simulink model "doc_concat"  (R2014a)
settings: Solver=ode45  SolverMode=SingleTasking  StartTime=0.0  StopTime=inf  RelTol=1e-3
values from neighbouring files (symbols this model uses):
  M = getTestParameter(obj,'M')    [GrayCodedMod_EbNo_M.m]    (also in GrayCodedModulation2.m; RSCodingConfigExample.m = 64; commdoc_bertool.m = 16; commdoc_code.m = 16)
undefined symbols (not defined in the file or in its folder): commblksprivate, EbNodB, Info, rsgenpoly
libraries: commutil2 x5, dspsigops x3, commcnvcod2 x2, commsink2 x2, commblkcod2 x2, commchan3 x1, commrandsrc2 x1
settings Model: Creator=The MathWorks Inc.
settings DataIOCC: SignalLoggingSaveFormat=ModelDataLogs  SaveOutput=off  SaveTime=off  SignalLoggingName=logsOut
settings OptimizationCC: BooleanDataType=off  InlineParams=on  ExpressionDepthLimit=2147483647  InitFltsAndDblsToZero=on
settings DebuggingCC: AlgebraicLoopMsg=error  SaveWithParameterizedLinksMsg=none  UnderspecifiedInitializationDetection=Classic  SignalResolutionControl=TryResolveAllWithWarning  SolverPrmCheckMsg=none  MultiTaskDSMMsg=warning  FcnCallInpInsideContextMsg=UseLocalSettings  StateNameClashWarn=warning  StrictBusMsg=None
settings HardwareCC: TargetUnknown=on
settings GRTTargetCC: TargetFcnLib=ansi_tfl_tmw.mat  CombineOutputUpdateFcns=off  GRTInterface=on

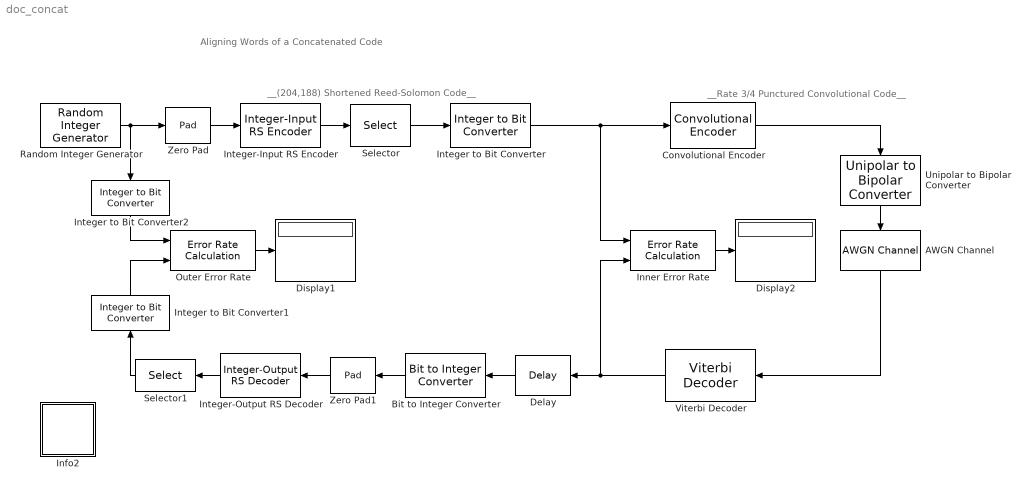
== system doc_concat ==
  note: __(204,188) Shortened Reed-Solomon Code__
  note: __Rate 3/4 Punctured Convolutional Code__
  note: Aligning Words of a Concatenated Code
  AWGN Channel : commchan3/AWGN Channel  InputProcessing=Columns as channels (frame based)  seed=68521  noiseMode="Signal to noise ratio  (SNR)"  EbNodB=10  EsNodB=EbNodB+10*log10(log2(M))  SNRdB=5  bitsPerSym=1  Ps=1  Tsym=Tsym  variance=10^(-0.1*15)/(2048*2)
  Bit to Integer Converter : commutil2/Bit to Integer Converter  nbits=8  bitOrder=MSB first  signedOutputValues=Unsigned  outDtype=Inherit via internal rule  outDtypeSigned=Inherit via internal rule
  Convolutional Encoder : commcnvcod2/Convolutional Encoder  trellis=poly2trellis(7, [171 133])  opMode=Continuous  DelayedResetAction=off  hasIniStPort=off  hasFinStPort=off  usePuncVector=on  punctureVector=[1 1 0 1 1 0]'  reset=Unused parameter value
  Delay : dspsigops/Delay  InputProcessing=Columns as channels (frame based)  dly_unit=Samples  delay=1632-136  ic_detail=off  dif_ic_for_ch=off  dif_ic_for_dly=off  ic=0  reset_popup=None
  Display1 : Display
  Display2 : Display
  Info2 : Subsystem  AncestorBlock=commblksprivate/Info  mask(Info){}
      settings: OpenFcn=helpview([docroot '/toolbox/comm/comm.map'], 'doc_concat')
      mask Display: disp('Info')
  Inner Error Rate : commsink2/Error Rate Calculation  N=136  st_delay=0  cp_mode=Entire frame  subframe=[]  PMode=Port  WsName=ErrorVec  RsMode2=off  stop=on  numErr=100  maxBits=1e6
  Integer to Bit Converter : commutil2/Integer to Bit Converter  nbits=8  signedInputValues=Unsigned  bitOrder=MSB first  outDtype=Inherit via internal rule
  Integer to Bit Converter1 : commutil2/Integer to Bit Converter  nbits=8  signedInputValues=Unsigned  bitOrder=MSB first  outDtype=Inherit via internal rule
  Integer to Bit Converter2 : commutil2/Integer to Bit Converter  nbits=8  signedInputValues=Unsigned  bitOrder=MSB first  outDtype=Inherit via internal rule
  Integer-Input RS Encoder : commblkcod2/Integer-Input RS Encoder  n=255  k=239  specPrimPoly=off  prPoly=[1 0 1 1]  specGenPoly=off  genPoly=rsgenpoly(7,3)  specPuncture=off  punctVec=[ones(2,1); zeros(2,1)]
  Integer-Output RS Decoder : commblkcod2/Integer-Output RS Decoder  n=255  k=239  specPrimPoly=off  prPoly=[1 0 1 1]  specGenPoly=off  genPoly=rsgenpoly(7,3)  specPuncture=off  punctVec=[ones(2,1); zeros(2,1)]  specErasurePort=off  showNumErr=off
  Outer Error Rate : commsink2/Error Rate Calculation  N=188*8  st_delay=0  cp_mode=Entire frame  subframe=[]  PMode=Port  WsName=ErrorVec  RsMode2=off  stop=off  numErr=100  maxBits=1e6
  Random Integer Generator : commrandsrc2/Random Integer Generator  mul=256  seed=56479  Ts=1  frameBased=on  sampPerFrame=188  orient=off  outDataType=double
  Selector : Selector  InputPortWidth=255  Indices=[1:204]
  Selector1 : Selector  InputPortWidth=239  Indices=[1:188]
  Unipolar to Bipolar Converter : commutil2/Unipolar to Bipolar Converter  M=2  polarity=Negative  dataType=Inherit via internal rule
  Viterbi Decoder : commcnvcod2/Viterbi Decoder  trellis=poly2trellis(7, [171 133])  isPunctured=on  punctureVector=[1 1 0 1 1 0]'  erasures=off  dectype=Unquantized  runSigValErrCheck=off  nsdecb=4  smWordLength=16  tbdepth=136  opmode=Continuous  reset=off  outDataType=double  delayedResetAction=off
  Zero Pad : dspsigops/Pad  padAlong=Columns  dimsToPad=1  valSrc=Specify via dialog  padVal=0  spec=Output size  padNumOutRowsSpecMethod=User-specified  numOutRows=239  padNumOutColsSpecMethod=User-specified  numOutCols=1  isVarDimsMode=off  padBeginning=0  padEnd=0  outSizeMode=User-specified  outSize=1  padSigAt=End  trunc_flag=None  roundingMode=Floor  overflowMode=off  truncOrWrapMode=Truncate  wrap_flag=None
  Zero Pad1 : dspsigops/Pad  padAlong=Columns  dimsToPad=1  valSrc=Specify via dialog  padVal=0  spec=Output size  padNumOutRowsSpecMethod=User-specified  numOutRows=255  padNumOutColsSpecMethod=User-specified  numOutCols=1  isVarDimsMode=off  padBeginning=0  padEnd=0  outSizeMode=User-specified  outSize=1  padSigAt=End  trunc_flag=None  roundingMode=Floor  overflowMode=off  truncOrWrapMode=Truncate  wrap_flag=None
  wires:
  Random Integer Generator/1 -> Zero Pad/1, Integer to Bit Converter2/1
  Zero Pad/1 -> Integer-Input RS Encoder/1
  Integer-Input RS Encoder/1 -> Selector/1
  Selector/1 -> Integer to Bit Converter/1
  Integer to Bit Converter/1 -> Inner Error Rate/1, Convolutional Encoder/1
  Convolutional Encoder/1 -> Unipolar to Bipolar Converter/1
  Bit to Integer Converter/1 -> Zero Pad1/1
  Zero Pad1/1 -> Integer-Output RS Decoder/1
  Integer-Output RS Decoder/1 -> Selector1/1
  Selector1/1 -> Integer to Bit Converter1/1
  Outer Error Rate/1 -> Display1/1
  Inner Error Rate/1 -> Display2/1
  Unipolar to Bipolar Converter/1 -> AWGN Channel/1
  Delay/1 -> Bit to Integer Converter/1
  AWGN Channel/1 -> Viterbi Decoder/1
  Integer to Bit Converter1/1 -> Outer Error Rate/2
  Integer to Bit Converter2/1 -> Outer Error Rate/1
  Viterbi Decoder/1 -> Delay/1, Inner Error Rate/2

== system doc_concat/Info2 ==
